simulink model "sim_proj1_timevar"  (R2022a)
settings: Solver=VariableStepAuto  StartTime=0.0  StopTime=1000  RelTol=1e-3
values from neighbouring files (symbols this model uses):
  sample = 1    [main_proj1.m]    (also in main_proj1_cheese.m)
undefined symbols (not defined in the file or in its folder): K
libraries: dspsrcs4 x7, cstblocks x1
settings Model: Creator=tikyn  LastModifiedBy=tikyn

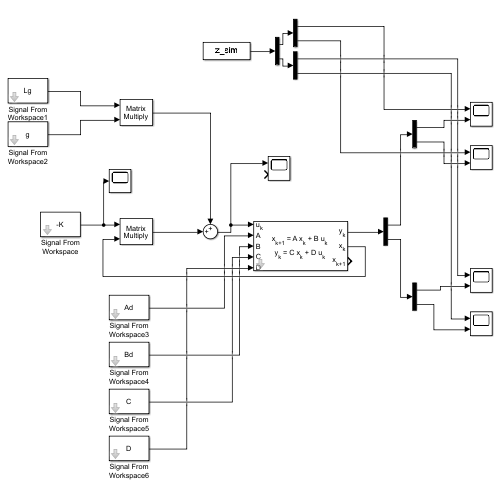
[thumbnail: Simulink's stored preview of the top-level diagram]
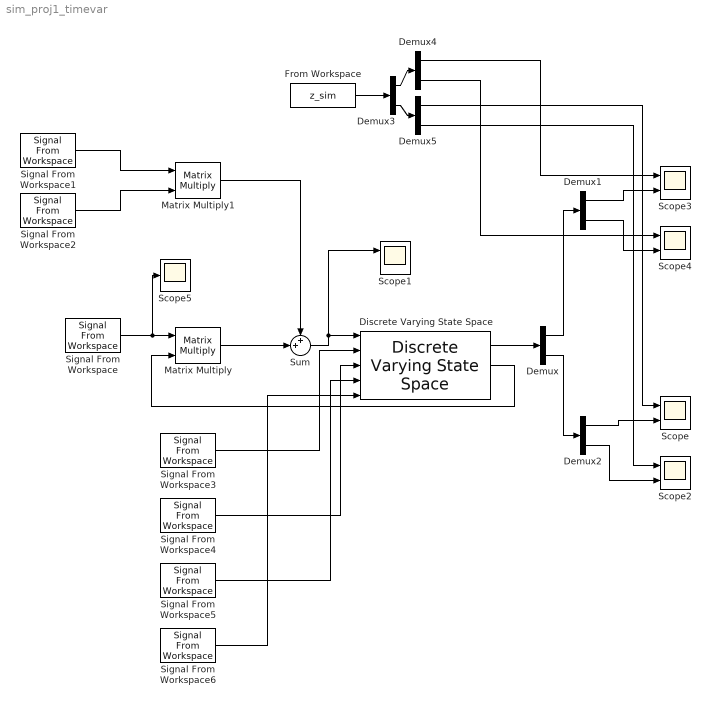
== system sim_proj1_timevar ==
  Demux{,1..5} (6 alike) : Demux  Outputs=2
  Discrete Varying State Space : cstblocks/Linear Parameter Varying/Discrete Varying State Space  x0=x_zero  Ts=sample  OutputX=on  OutputDX=on
      settings: SourceProductBaseCode=CT
  From Workspace : FromWorkspace  VariableName=z_sim  SampleTime=1
  Matrix Multiply : Product  Multiplication=Matrix(*)
  Matrix Multiply1 : Product  Multiplication=Matrix(*)
  Scope{,1..4} (5 alike) : Scope  NumInputPorts=2
  Scope5 : Scope
  Signal From Workspace : dspsrcs4/Signal From Workspace  X=-K  Ts=1  nsamps=1  OutputAfterFinalValue=Setting to zero  ignoreOrWarnInputAndFrameLengths=off  OutputFrames=off
  Signal From Workspace1 : dspsrcs4/Signal From Workspace  X=Lg  Ts=1  nsamps=1  OutputAfterFinalValue=Setting to zero  ignoreOrWarnInputAndFrameLengths=off  OutputFrames=off
  Signal From Workspace2 : dspsrcs4/Signal From Workspace  X=g  Ts=1  nsamps=1  OutputAfterFinalValue=Setting to zero  ignoreOrWarnInputAndFrameLengths=off  OutputFrames=off
  Signal From Workspace3 : dspsrcs4/Signal From Workspace  X=Ad  Ts=1  nsamps=1  OutputAfterFinalValue=Setting to zero  ignoreOrWarnInputAndFrameLengths=off  OutputFrames=off
  Signal From Workspace4 : dspsrcs4/Signal From Workspace  X=Bd  Ts=1  nsamps=1  OutputAfterFinalValue=Setting to zero  ignoreOrWarnInputAndFrameLengths=off  OutputFrames=off
  Signal From Workspace5 : dspsrcs4/Signal From Workspace  X=C  Ts=1  nsamps=1  OutputAfterFinalValue=Setting to zero  ignoreOrWarnInputAndFrameLengths=off  OutputFrames=off
  Signal From Workspace6 : dspsrcs4/Signal From Workspace  X=D  Ts=1  nsamps=1  OutputAfterFinalValue=Setting to zero  ignoreOrWarnInputAndFrameLengths=off  OutputFrames=off
  Sum : Sum  Inputs=++|
  wires:
  Demux1/2 -> Scope4/2
  Demux2/2 -> Scope2/2
  Demux/1 -> Demux1/1
  Signal From Workspace1/1 -> Matrix Multiply1/1
  Demux/2 -> Demux2/1
  Signal From Workspace/1 -> Scope5/1, Matrix Multiply/1
  Sum/1 -> Scope1/1, Discrete Varying State Space/1
  Demux2/1 -> Scope/2
  Matrix Multiply1/1 -> Sum/1
  Discrete Varying State Space/1 -> Demux/1
  Demux1/1 -> Scope3/2
  Signal From Workspace2/1 -> Matrix Multiply1/2
  Matrix Multiply/1 -> Sum/2
  Signal From Workspace3/1 -> Discrete Varying State Space/2
  Signal From Workspace4/1 -> Discrete Varying State Space/3
  Signal From Workspace5/1 -> Discrete Varying State Space/4
  Signal From Workspace6/1 -> Discrete Varying State Space/5
  Discrete Varying State Space/2 -> Matrix Multiply/2
  Demux3/1 -> Demux4/1
  Demux3/2 -> Demux5/1
  From Workspace/1 -> Demux3/1
  Demux4/1 -> Scope3/1
  Demux4/2 -> Scope4/1
  Demux5/1 -> Scope/1
  Demux5/2 -> Scope2/1
